simulink model "bus_roadtest_v3"  (R2018a)
settings: Solver=ode3  StartTime=0.0  StopTime=inf  FixedStep=0.01  RelTol=1e-3  EnableMultiTasking=on
PostLoadFcn:
  | , if any(exist('dsrtsu_mdlpostloadfcn', 'file') == [2, 3, 6]), try dsrtsu_mdlpostloadfcn('Execute', bdroot); catch fprintf('Error in PostLoadFcn (dsrtsu_mdlpostloadfcn) for model "%s":\n %s\n', bdroot, lasterr); end, end,
InitFcn:
  | bus_roadtest_v3_initial
values from neighbouring files (symbols this model uses):
  ay_max = 2    [Ini.m]
  delta_t = 0.01    [Ini.m]
  end_left_pass = 1    [Ini.m]
  end_right_pass = 0    [Ini.m]
  finish_node_id = length(Map_data(:,1))    [Ini.m]
  forward_length = 15    [Ini.m]
  gamma = sqrt(N_xaug+lambda)    [bus_roadtest_v3_initial.m]
  k_safe = 1    [Ini.m]
  nodes = nodes(1:index_node,:)    [Ini.m]
  rmin = 10    [Ini.m]
  segments = zeros(length(xy_ends_Pos(:,1)),3)    [Ini.m]
  start_node_id = 1    [Ini.m]
  Ts = 0.01    [bus_roadtest_v3_initial.m]
  Veh_CG = [0.5, 0.2]    [Ini.m]
  Veh_size = [1.99986,6.09558]    [Ini.m]
  vmax = 6    [Ini.m]
  weight = [weight_0,weight_0_cov,weight_i]    [bus_roadtest_v3_initial.m]
undefined symbols (not defined in the file or in its folder): Brake_table, DiscIntNeverNeededParam, Map_data, R, REF_GPS_RFS, Steer_gain_table, T
libraries: rtican x71, simulink x26, rti1401lib_adc_type4 x8, rti1401lib_dio_type4 x1
(part 14 of 18)

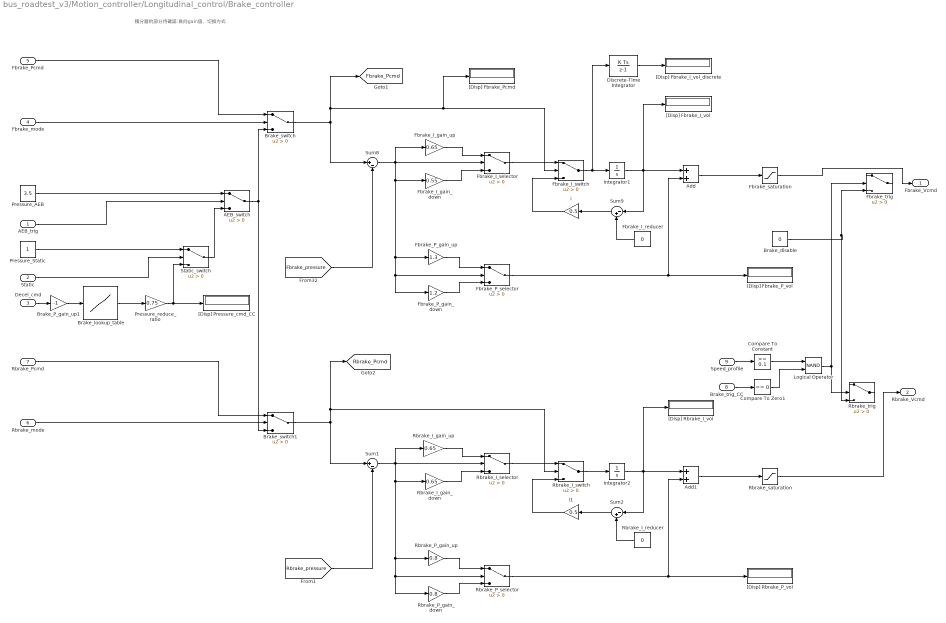
== system bus_roadtest_v3/Motion_controller/Longitudinal_control/Brake_controller ==
  note: 積分器的部分待確認:負向gain值、切換方式
  AEB_trig : Inport
  Static : Inport  Port=2
  Decel_cmd : Inport  Port=3
  Fbrake_mode : Inport  Port=4
  Fbrake_Pcmd : Inport  Port=5
  Rbrake_mode : Inport  Port=6
  Rbrake_Pcmd : Inport  Port=7
  Brake_trig_CC : Inport  Port=8
  Speed_profile : Inport  Port=9
  AEB_switch : Switch  Criteria=u2 > Threshold
  Add : Sum
  Add1 : Sum
  Brake_P_gain_up1 : Gain  Gain=-1
  Brake_disable : Constant  Value=0
  Brake_lookup_table : Lookup_n-D  NumberOfTableDimensions=1  BreakpointsForDimension1=Brake_table(2,:)  Table=Brake_table(1,:)  InterpMethod=Flat  InternalRulePriority=Speed  RndMeth=Simplest  InputSameDT=on
  Brake_switch : Switch  Criteria=u2 > Threshold
  Brake_switch1 : Switch  Criteria=u2 > Threshold
  Compare To Constant : simulink/Logic and Bit Operations/Compare To Constant  relop=>=  const=0.1  OutDataTypeStr=boolean
  Compare To Zero1 : simulink/Logic and Bit Operations/Compare To Zero  relop===  OutDataTypeStr=boolean
  Discrete-Time Integrator : DiscreteIntegrator  SampleTime=0.01  LimitOutput=on  UpperSaturationLimit=5  LowerSaturationLimit=-100  ICPrevOutput=DiscIntNeverNeededParam  ICPrevScaledInput=DiscIntNeverNeededParam
  Fbrake_I_gain_down : Gain  Gain=0.55
  Fbrake_I_gain_up : Gain  Gain=0.65
  Fbrake_I_reducer : Constant  Value=0
  Fbrake_I_selector : Switch  Criteria=u2 > Threshold
  Fbrake_I_switch : Switch  Criteria=u2 > Threshold
  Fbrake_P_gain_down : Gain  Gain=1.2
  Fbrake_P_gain_up : Gain  Gain=1.3
  Fbrake_P_selector : Switch  Criteria=u2 > Threshold
  Fbrake_saturation : Saturate  UpperLimit=4.8  LowerLimit=0
  Fbrake_trig : Switch  Criteria=u2 > Threshold
  Integrator1 : Integrator  LimitOutput=on  UpperSaturationLimit=5  LowerSaturationLimit=-100
  Integrator2 : Integrator  LimitOutput=on  UpperSaturationLimit=5  LowerSaturationLimit=-100
  Logical Operator : Logic  Operator=NAND  AllPortsSameDT=off  OutDataTypeStr=boolean
  Pressure_AEB : Constant  Value=3.5
  Pressure_Static : Constant
  Pressure_reduce_ratio : Gain  Gain=0.75
  Rbrake_I_gain_down : Gain  Gain=0.65
  Rbrake_I_gain_up : Gain  Gain=0.65
  Rbrake_I_reducer : Constant  Value=0
  Rbrake_I_selector : Switch  Criteria=u2 > Threshold
  Rbrake_I_switch : Switch  Criteria=u2 > Threshold
  Rbrake_P_gain_down : Gain  Gain=0.8
  Rbrake_P_gain_up : Gain  Gain=0.8
  Rbrake_P_selector : Switch  Criteria=u2 > Threshold
  Rbrake_saturation : Saturate  UpperLimit=4.8  LowerLimit=0
  Rbrake_trig : Switch  Criteria=u2 > Threshold
  Static_switch : Switch  Criteria=u2 > Threshold
  Sum1 : Sum  Inputs=|+-
  Sum2 : Sum  Inputs=|-+
  Sum8 : Sum  Inputs=|+-
  Sum9 : Sum  Inputs=|-+
  "[Disp] Fbrake_I_vol" : Display
  "[Disp] Fbrake_I_vol_discrete" : Display
  "[Disp] Fbrake_P_vol" : Display
  "[Disp] Fbrake_Pcmd" : Display
  "[Disp] Pressure_cmd_CC" : Display
  "[Disp] Rbrake_I_vol" : Display
  "[Disp] Rbrake_P_vol" : Display
  i : Gain  Gain=0.5
  i1 : Gain  Gain=0.5
  Fbrake_Vcmd : Outport
  Rbrake_Vcmd : Outport  Port=2
  tag scope: Fbrake_Pcmd=global, Rbrake_Pcmd=global
  wires:
  Fbrake_I_gain_up/1 -> Fbrake_I_selector/1
  Fbrake_P_selector/1 -> "[Disp] Fbrake_P_vol"/1, Add/2
  Integrator1/1 -> Add/1, "[Disp] Fbrake_I_vol"/1, Sum9/1
  Sum8/1 -> Fbrake_I_gain_up/1, Fbrake_I_selector/2, Fbrake_P_selector/2, Fbrake_P_gain_down/1, Fbrake_P_gain_up/1, Fbrake_I_gain_down/1
  Fbrake_I_gain_down/1 -> Fbrake_I_selector/3
  Fbrake_P_gain_up/1 -> Fbrake_P_selector/1
  Fbrake_P_gain_down/1 -> Fbrake_P_selector/3
  AEB_trig/1 -> AEB_switch/2
  Pressure_AEB/1 -> AEB_switch/1
  Static_switch/1 -> AEB_switch/3
  Pressure_Static/1 -> Static_switch/1
  Brake_lookup_table/1 -> Pressure_reduce_ratio/1
  [Fbrake_pressure] -> Sum8/2
  Fbrake_I_reducer/1 -> Sum9/2
  Sum9/1 -> i/1
  Fbrake_I_switch/1 -> Discrete-Time Integrator/1, Integrator1/1
  Fbrake_I_selector/1 -> Fbrake_I_switch/1
  i/1 -> Fbrake_I_switch/3
  Decel_cmd/1 -> Brake_P_gain_up1/1
  Brake_P_gain_up1/1 -> Brake_lookup_table/1
  Static/1 -> Static_switch/2
  Fbrake_mode/1 -> Brake_switch/2
  Brake_switch/1 -> [Fbrake_Pcmd], "[Disp] Fbrake_Pcmd"/1, Fbrake_I_switch/2, Sum8/1
  Fbrake_Pcmd/1 -> Brake_switch/1
  Rbrake_Pcmd/1 -> Brake_switch1/1
  Brake_switch1/1 -> Sum1/1, [Rbrake_Pcmd], Rbrake_I_switch/2
  Rbrake_mode/1 -> Brake_switch1/2
  i1/1 -> Rbrake_I_switch/3
  Rbrake_I_selector/1 -> Rbrake_I_switch/1
  Rbrake_I_switch/1 -> Integrator2/1
  Sum2/1 -> i1/1
  Rbrake_I_reducer/1 -> Sum2/2
  [Rbrake_pressure] -> Sum1/2
  Rbrake_P_gain_down/1 -> Rbrake_P_selector/3
  Rbrake_P_gain_up/1 -> Rbrake_P_selector/1
  Rbrake_I_gain_down/1 -> Rbrake_I_selector/3
  Sum1/1 -> Rbrake_I_gain_down/1, Rbrake_P_gain_up/1, Rbrake_P_gain_down/1, Rbrake_P_selector/2, Rbrake_I_selector/2, Rbrake_I_gain_up/1
  Integrator2/1 -> Sum2/1, "[Disp] Rbrake_I_vol"/1, Add1/1
  Rbrake_P_selector/1 -> Add1/2, "[Disp] Rbrake_P_vol"/1
  Rbrake_I_gain_up/1 -> Rbrake_I_selector/1
  Add/1 -> Fbrake_saturation/1
  Add1/1 -> Rbrake_saturation/1
  AEB_switch/1 -> Brake_switch1/3, Brake_switch/3
  Pressure_reduce_ratio/1 -> "[Disp] Pressure_cmd_CC"/1, Static_switch/3
  Brake_disable/1 -> Rbrake_trig/3, Fbrake_trig/3
  Speed_profile/1 -> Compare To Constant/1
  Brake_trig_CC/1 -> Compare To Zero1/1
  Compare To Constant/1 -> Logical Operator/1
  Compare To Zero1/1 -> Logical Operator/2
  Logical Operator/1 -> Fbrake_trig/2, Rbrake_trig/2
  Discrete-Time Integrator/1 -> "[Disp] Fbrake_I_vol_discrete"/1
  Rbrake_saturation/1 -> Rbrake_Vcmd/1
  Fbrake_saturation/1 -> Fbrake_Vcmd/1

== system bus_roadtest_v3/Motion_controller/Longitudinal_control/Switching_module ==
  AEB_trig : Inport
  Static : Inport  Port=2
  Speed_profile : Inport  Port=3
  Brake_trig_CC_status : Inport  Port=4
  Base_decel : Constant  Value=0.2
  Brake_Throttle_toggle : MATLAB Function  TreatAsAtomicUnit=on
  Brake_lock_on : Constant
  Brake_status : MATLAB Function  TreatAsAtomicUnit=on
  Brake_trig_bound : Saturate  UpperLimit=-0.2  LowerLimit=-5
  Brake_trig_shreshold : simulink/Logic and Bit Operations/Compare To Constant  relop=<=  const=-0.8  OutDataTypeStr=boolean
  Compare To Constant : simulink/Logic and Bit Operations/Compare To Constant  relop=>=  const=0.5  OutDataTypeStr=boolean
  Compare To Constant1 : simulink/Logic and Bit Operations/Compare To Constant  relop=>=  const=0.5  OutDataTypeStr=boolean
  Constant : Constant  Value=0
  Constant1 : Constant  Value=100
  Constant2 : Constant  Value=10
  Constant3 : Constant  Value=0.25
  Constant4 : Constant  Value=0.2
  Discrete Transfer Fcn : DiscreteTransferFcn  Numerator=[0.09516]  Denominator=[1 -0.9048]
  Logical Operator : Logic  Operator=OR  Inputs=4  AllPortsSameDT=off  OutDataTypeStr=boolean
  Logical Operator1 : Logic  Operator=OR  AllPortsSameDT=off  OutDataTypeStr=boolean
  Logical Operator2 : Logic  Operator=OR  AllPortsSameDT=off  OutDataTypeStr=boolean
  Logical Operator3 : Logic  AllPortsSameDT=off  OutDataTypeStr=boolean
  MATLAB Function : MATLAB Function  TreatAsAtomicUnit=on
  Relational Operator : RelationalOperator  Operator=>  OutDataTypeStr=boolean  RndMeth=Simplest
  Speed_err_gain : Gain
  Sum : Sum  Inputs=|+-
  Sum1 : Sum  Inputs=|+-
  Switch : Switch  Criteria=u2 > Threshold
  Switch1 : Switch  Criteria=u2 > Threshold
  Switch2 : Switch  Criteria=u2 > Threshold
  Transfer Fcn : TransferFcn  Numerator=[10]  Denominator=[1 10]
  "[Disp] Accel_err" : Display
  "[Disp] Accel_err_discrete" : Display
  "[Disp] Brake_status" : Display
  "[Disp] Brake_trig_CC" : Display
  "[Disp] Decel_cmd" : Display
  "[Disp] Speed_err" : Display
  "[Disp] Throttle_resume" : Display
  kph2mps : Gain  Gain=1/3.6
  Speed_cmd : Outport
  Decel_cmd : Outport  Port=2
  Brake_trig_CC : Outport  Port=3
  tag scope: Brake_status=global, Brake_trig_CC=global
  wires:
  Speed_profile/1 -> Sum/1, Switch/3
  [Speed_Kph] -> MATLAB Function/1(Speed_cmd), Sum/2
  Sum/1 -> kph2mps/1
  kph2mps/1 -> Speed_err_gain/1, "[Disp] Speed_err"/1
  Brake_Throttle_toggle/1(Brake_trig_CC) -> Logical Operator/3, Switch1/2, Brake_status/3(CC_trig), Brake_trig_CC/1, [Brake_trig_CC], "[Disp] Brake_trig_CC"/1
  Brake_trig_shreshold/1 -> Brake_Throttle_toggle/1(B_toggle)
  Relational Operator/1 -> Brake_Throttle_toggle/2(T_toggle)
  Brake_trig_CC_status/1 -> Brake_Throttle_toggle/3(Last_status)
  Switch/1 -> Speed_cmd/1
  Constant/1 -> Switch1/3, Switch/1
  AEB_trig/1 -> Logical Operator/1, Brake_status/1(AEB), Logical Operator1/1
  Static/1 -> Brake_status/2(Static), Logical Operator/2, Logical Operator1/2, Brake_Throttle_toggle/4(Static_flag)
  Logical Operator/1 -> Switch/2
  Switch2/1 -> "[Disp] Decel_cmd"/1, Decel_cmd/1
  Logical Operator1/1 -> Switch2/2
  Switch1/1 -> Switch2/3
  Constant1/1 -> Switch2/1
  Speed_err_gain/1 -> Discrete Transfer Fcn/1, Transfer Fcn/1
  Sum1/1 -> Brake_trig_bound/1
  Transfer Fcn/1 -> "[Disp] Accel_err"/1, Sum1/1, Relational Operator/1, Brake_trig_shreshold/1
  Base_decel/1 -> Sum1/2
  Brake_trig_bound/1 -> Switch1/1
  Constant2/1 -> MATLAB Function/2(Speed_bound)
  Constant3/1 -> MATLAB Function/3(upper_ratio)
  Constant4/1 -> MATLAB Function/4(lower_ratio)
  MATLAB Function/1(T_resume) -> "[Disp] Throttle_resume"/1, Relational Operator/2
  [Fbrake_pressure] -> Compare To Constant/1
  [Rbrake_pressure] -> Compare To Constant1/1
  Compare To Constant1/1 -> Logical Operator2/2
  Compare To Constant/1 -> Logical Operator2/1
  Logical Operator2/1 -> Logical Operator3/2
  Logical Operator3/1 -> Logical Operator/4
  Brake_lock_on/1 -> Logical Operator3/1
  Discrete Transfer Fcn/1 -> "[Disp] Accel_err_discrete"/1
  [Fbrake_interrupt] -> Brake_status/4(interrupt)
  Brake_status/1(Brake_status) -> [Brake_status], "[Disp] Brake_status"/1

== system bus_roadtest_v3/Motion_controller/Longitudinal_control/Throttle_controller ==
  Throttle_mode : Inport
  Throttle_vol : Inport  Port=2
  AEB_trig : Inport  Port=3
  Static : Inport  Port=4
  Speed_cmd : Inport  Port=5
  AEB_switch_T : Switch  Criteria=u2 > Threshold
  Constant : Constant  Value=0
  I_gain_windup : Switch  Criteria=u2 > Threshold
  I_gain_windup1 : Switch  Criteria=u2 > Threshold
  I_windup_limit : simulink/Logic and Bit Operations/Compare To Constant  relop=<=  const=2  OutDataTypeStr=boolean
  I_windup_on : Constant
  Logical Operator : Logic  Operator=OR  AllPortsSameDT=off  OutDataTypeStr=boolean
  Sum1 : Sum  Inputs=|++
  Sum2 : Sum  Inputs=|+-
  Sum3 : Sum  Inputs=|+-
  Sum4 : Sum  Inputs=+|+
  Sum6 : Sum  Inputs=|++
  Sum7 : Sum  Inputs=|+-
  Throttle_I_gain : Gain  Gain=0.05
  Throttle_I_gain_down : Gain  Gain=0.05
  Throttle_I_integrator : Integrator  LimitOutput=on  UpperSaturationLimit=4.68  LowerSaturationLimit=0
  Throttle_I_reducer : Constant  Value=0
  Throttle_I_saturation : Saturate  UpperLimit=2  LowerLimit=0
  Throttle_I_switch : Switch  Criteria=u2 > Threshold
  Throttle_I_switch1 : Switch  Criteria=u2 > Threshold
  Throttle_P_gain : Gain  Gain=0.2
  Throttle_boost_on : Constant
  Throttle_boost_vol : Constant  Value=0.8
  Throttle_boost_zero : Constant  Value=0
  Throttle_saturation : Saturate  UpperLimit=4.68  LowerLimit=0.04
  Throttle_switch : Switch  Criteria=u2 > Threshold
  Throttle_switch1 : Switch  Criteria=u2 > Threshold
  Throttle_switch2 : Switch  Criteria=u2 > Threshold
  "[Disp] Speed_cmd_controller" : Display
  "[Disp] Throttle_I_vol" : Display
  "[Disp] Throttle_I_windup" : Display
  "[Disp] Throttle_P_vol" : Display
  "[Disp] Throttle_T_vol" : Display
  "[Disp] Throttle_boost_vol" : Display
  speed P gain1 : Gain  Gain=0.5
  Throttle_out : Outport
  wires:
  Throttle_vol/1 -> Throttle_switch/1
  Sum2/1 -> Throttle_P_gain/1, Throttle_I_gain_down/1, Throttle_I_switch1/2, Throttle_I_gain/1
  Throttle_P_gain/1 -> "[Disp] Throttle_P_vol"/1, Sum6/1
  Throttle_I_integrator/1 -> Sum3/2, Sum7/2, Throttle_I_saturation/1, Sum6/2, "[Disp] Throttle_I_vol"/1
  Throttle_I_switch/1 -> Throttle_I_integrator/1
  Throttle_I_reducer/1 -> Sum7/1, I_gain_windup1/3, I_gain_windup/1
  Sum7/1 -> speed P gain1/1
  speed P gain1/1 -> Throttle_I_switch/3
  Throttle_saturation/1 -> "[Disp] Throttle_T_vol"/1, Throttle_switch/3
  Speed_cmd/1 -> Sum2/1, "[Disp] Speed_cmd_controller"/1, Throttle_switch2/2, Throttle_I_switch/2
  [Speed_Kph] -> Sum2/2
  AEB_trig/1 -> Logical Operator/1
  Static/1 -> Logical Operator/2
  Throttle_switch/1 -> AEB_switch_T/3
  AEB_switch_T/1 -> Throttle_out/1
  Logical Operator/1 -> AEB_switch_T/2
  Constant/1 -> AEB_switch_T/1
  Throttle_mode/1 -> Throttle_switch/2
  Throttle_boost_vol/1 -> Throttle_switch2/1
  Throttle_boost_on/1 -> Throttle_switch1/2
  Throttle_boost_zero/1 -> Throttle_switch2/3, Throttle_switch1/3
  Sum6/1 -> Sum1/1
  Sum1/1 -> Throttle_saturation/1
  Throttle_switch1/1 -> "[Disp] Throttle_boost_vol"/1, Sum1/2
  Throttle_switch2/1 -> Throttle_switch1/1
  Throttle_I_gain/1 -> Throttle_I_switch1/1
  Throttle_I_gain_down/1 -> Throttle_I_switch1/3
  Throttle_I_saturation/1 -> Sum3/1
  Sum3/1 -> I_gain_windup/3
  Throttle_I_switch1/1 -> Sum4/1
  Sum4/1 -> Throttle_I_switch/1
  [Speed_Kph] -> I_windup_limit/1
  I_windup_limit/1 -> I_gain_windup/2
  I_windup_on/1 -> I_gain_windup1/2
  I_gain_windup1/1 -> "[Disp] Throttle_I_windup"/1, Sum4/2
  I_gain_windup/1 -> I_gain_windup1/1

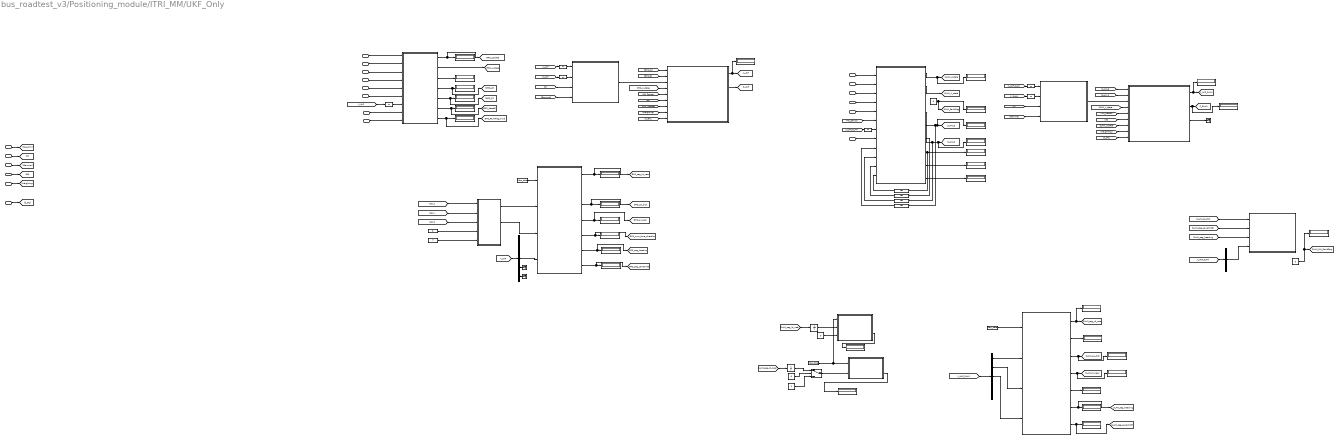
== system bus_roadtest_v3/Positioning_module/ITRI_MM/UKF_Only ==
  note: 建立取樣點UKF(對照組)
  note: 建立取樣點UKF_SLAM
  note: MM線段:得知當下最近道路，得知道路資訊
  note: GNSS模組
  note: GNSS Check
  note: GNSS MM
  note: SLAM模組
  note: SLAM Check
  note: SLAM UKF
  note: SLAM UKF MM
  note: SLAM UKF MM Check模組
  GPS_X : Inport
  GPS_Y : Inport  Port=2
  GPS_Heading : Inport  Port=3
  Road _Alt_GPS : Inport  Port=4
  IMU : Inport  Port=5
  Sig_dim : Inport  Port=6
  N : Inport  Port=7
  Gamma : Inport  Port=8
  dt : Inport  Port=9
  weighting : Inport  Port=10
  GPS_TYPE : Inport  Port=11
  GPS_X_ACC : Inport  Port=12
  GPS_Y_ACC : Inport  Port=13
  d_GC : Inport  Port=14
  SLAM_X : Inport  Port=15
  SLAM_Y : Inport  Port=16
  SLAM_Heading : Inport  Port=17
  SLAM_Counter : Inport  Port=18
  SLAM_FS : Inport  Port=19
  SLAM_fault : Inport  Port=20
  Constant : Constant  Value=0
  Constant1 : Constant  Value=Map_data
  Constant2 : Constant  Value=T
  Constant22 : Constant  Value=Map_data
  Constant29 : Constant  Value=R
  Constant3 : Constant  Value=0
  Constant4 : Constant  Value=Map_data
  Demux : Demux  Outputs=5
  Demux1 : Demux  Outputs=5
  Demux2 : Demux  Outputs=5
  ENU2SLAM : MATLAB Function  TreatAsAtomicUnit=on
  GNSS_Check : Subsystem
  GNSS_UKF : MATLAB Function  TreatAsAtomicUnit=on
  GNSS_UKF_MM : MATLAB Function  TreatAsAtomicUnit=on
  Generate_sigma_pt_UKF : MATLAB Function  TreatAsAtomicUnit=on
  MATLAB Function : MATLAB Function  TreatAsAtomicUnit=on
  MATLAB Function1 : MATLAB Function  TreatAsAtomicUnit=on
  SLAM_Check : MATLAB Function  TreatAsAtomicUnit=on
  SLAM_Generate_sigma_pt_UKF : MATLAB Function  TreatAsAtomicUnit=on
  SLAM_UKF : MATLAB Function  TreatAsAtomicUnit=on
  SLAM_UKF_MM : MATLAB Function  TreatAsAtomicUnit=on
  SLAM_UKF_MM_Check : MATLAB Function  TreatAsAtomicUnit=on
  Switch : Switch  Criteria=u2 > Threshold
  Terminator2 : Terminator
  Terminator3 : Terminator
  Terminator5 : Terminator
  Unit Delay : UnitDelay  InitialCondition=1  SampleTime=-1
  Unit Delay{1,9,14,34} (4 alike) : UnitDelay  InitialCondition=[0;0;0;0;0]  SampleTime=-1
  Unit Delay10 : UnitDelay  InitialCondition=[eye(5)*0.001]  SampleTime=-1
  Unit Delay2 : UnitDelay  InitialCondition=1  SampleTime=-1
  Unit Delay33 : UnitDelay  InitialCondition=[eye(5)*0.001]  SampleTime=-1
  Unit Delay35 : UnitDelay  InitialCondition=[0,0,0,0]  SampleTime=-1
  Unit Delay36 : UnitDelay  InitialCondition=diag([0.1,0.1,0.1,0.0001,0.0001])  SampleTime=-1
  Unit Delay37 : UnitDelay  InitialCondition=diag([0.00025,0.00025,0.0000001,1,0.0001])  SampleTime=-1
  Unit Delay38 : UnitDelay  SampleTime=-1
  "[Disp] Forward_segid" : Display
  "[Disp] Forward_segid1" : Display
  "[Disp] GPS_FaultFlag" : Display
  "[Disp] GPS_FaultFlag_True" : Display
  "[Disp] GPS_Q" : Display
  "[Disp] GPS_R" : Display
  "[Disp] GPS_ResetP" : Display
  "[Disp] GPS_Update_UKF" : Display
  "[Disp] GPS_num_lane_direction" : Display
  "[Disp] GPS_oi_near" : Display
  "[Disp] GPS_op_dist" : Display
  "[Disp] GPS_seg_LaneWidth" : Display
  "[Disp] GPS_seg_heading" : Display
  "[Disp] GPS_seg_id_near" : Display
  "[Disp] P_SLAM" : Display
  "[Disp] SLAM_FaultFalg" : Display
  "[Disp] SLAM_FaultFlag_case" : Display
  "[Disp] SLAM_MM_FaultFlag" : Display
  "[Disp] SLAM_Q" : Display
  "[Disp] SLAM_R" : Display
  "[Disp] SLAM_dist_op" : Display
  "[Disp] SLAM_num_lane_direction" : Display
  "[Disp] SLAM_oi_near" : Display
  "[Disp] SLAM_op_dist" : Display
  "[Disp] SLAM_seg_LaneWidth" : Display
  "[Disp] SLAM_seg_heading" : Display
  "[Disp] SLAM_seg_id_near" : Display
  "[Disp] SLAM_update" : Display
  "[Disp] SLAM_update_count" : Display
  "[Disp] X_UKF" : Display
  "[Disp] X_UKF_SLAM" : Display
  "[Disp] dist_SLAMlastUKFSLAM" : Display
  "[Para] Inisegid" : Constant
  "[Para] Inisegswitch" : Constant  Value=0
  "[Para] Map_switch" : Constant  Value=0
  tag scope: GPS_FaultFlag_True=global, GPS_Update=global, GPS_X_state=global, GPS_num_lane_direction=global, GPS_oi_near=global, GPS_op_dist=global, GPS_seg_LaneWidth=global, GPS_seg_heading=global, GPS_seg_id_near=global, P_SLAM=global, P_UKF=global, SLAM_FaultFlag=global, SLAM_MM_FaultFlag=global, SLAM_Q=global, SLAM_R=global, SLAM_X_state=global, SLAM_oi_near=global, SLAM_op_dist=global, SLAM_seg_LaneWidth=global, SLAM_seg_heading=global, SLAM_seg_id_near=global, SLAM_update=global, X_UKF=global, X_UKF_SLAM=global
  wires:
  GNSS_Check/1(GPS_update) -> [GPS_Update], "[Disp] GPS_Update_UKF"/1
  GNSS_Check/2(X_state) -> [GPS_X_state]
  Sig_dim/1 -> [Sig_dim]
  N/1 -> [N]
  Gamma/1 -> [Gamma]
  dt/1 -> [dt]
  weighting/1 -> [weighting]
  Unit Delay10/1 -> Generate_sigma_pt_UKF/2(IC_P)
  Unit Delay9/1 -> Generate_sigma_pt_UKF/1(IC_X)
  [X_UKF] -> Unit Delay9/1
  [P_UKF] -> Unit Delay10/1
  [N] -> Generate_sigma_pt_UKF/3(n)
  [Gamma] -> Generate_sigma_pt_UKF/4(gamma)
  GPS_X/1 -> GNSS_Check/1(GPS_X)
  GPS_Y/1 -> GNSS_Check/2(GPS_Y)
  GPS_Heading/1 -> GNSS_Check/3(GPS_Heading)
  Road _Alt_GPS/1 -> GNSS_Check/4(Road_Alt_GPS)
  IMU/1 -> GNSS_Check/5(IMU)
  GPS_TYPE/1 -> GNSS_Check/6(GPS_TYPE)
  GNSS_Check/4(Q_last_o) -> [GPS_Q], "[Disp] GPS_Q"/1
  GNSS_Check/5(R_last_o) -> [GPS_R], "[Disp] GPS_R"/1
  [X_UKF] -> Unit Delay14/1
  Unit Delay14/1 -> GNSS_Check/7(X_UKF)
  GNSS_Check/3(GNSS_FaultFlag) -> "[Disp] GPS_FaultFlag"/1
  GNSS_Check/6(ResetP) -> [GPS_ResetP], "[Disp] GPS_ResetP"/1
  GPS_X_ACC/1 -> GNSS_Check/8(GPS_X_Acc)
  GPS_Y_ACC/1 -> GNSS_Check/9(GPS_Y_Acc)
  d_GC/1 -> [d_GC]
  [X_UKF] -> Demux/1
  Demux/4 -> Terminator2/1
  Demux/5 -> Terminator3/1
  [N] -> SLAM_Generate_sigma_pt_UKF/3(n)
  [Gamma] -> SLAM_Generate_sigma_pt_UKF/4(gamma)
  SLAM_Generate_sigma_pt_UKF/1(X_AUG) -> SLAM_UKF/3(X_AUG)
  [SLAM_X_state] -> SLAM_UKF/4(X_state)
  [SLAM_update] -> SLAM_UKF/7(SLAM_update)
  [dt] -> SLAM_UKF/6(Sensor_dt)
  [IMU_Sensor] -> SLAM_UKF/5(IMU_Sensor)
  [weighting] -> SLAM_UKF/8(weighting)
  SLAM_UKF/1(X) -> "[Disp] X_UKF_SLAM"/1, [X_UKF_SLAM]
  SLAM_UKF/2(P) -> "[Disp] P_SLAM"/1, [P_SLAM]
  SLAM_UKF/3(K) -> Terminator5/1
  Unit Delay33/1 -> SLAM_Generate_sigma_pt_UKF/2(IC_P)
  Unit Delay34/1 -> SLAM_Generate_sigma_pt_UKF/1(IC_X)
  [X_UKF_SLAM] -> Unit Delay34/1
  [P_SLAM] -> Unit Delay33/1
  SLAM_UKF_MM/3(op_distance) -> "[Disp] SLAM_op_dist"/1, [SLAM_op_dist]
  SLAM_UKF_MM/1(seg_id_near) -> "[Disp] SLAM_seg_id_near"/1, [SLAM_seg_id_near]
  SLAM_UKF_MM/4(Oi_near) -> "[Disp] SLAM_oi_near"/1, [SLAM_oi_near]
  [SLAM_R] -> SLAM_UKF/2(R)
  SLAM_UKF_MM/5(num_lane_direction) -> "[Disp] SLAM_num_lane_direction"/1
  [SLAM_Q] -> SLAM_UKF/1(Q)
  [d_GC] -> SLAM_UKF/9(d_GC)
  SLAM_X/1 -> SLAM_Check/2(SLAM_X)
  SLAM_Y/1 -> SLAM_Check/3(SLAM_Y)
  SLAM_Heading/1 -> SLAM_Check/4(SLAM_Heading)
  SLAM_Counter/1 -> SLAM_Check/5(SLAM_Counter)
  [IMU_Sensor] -> SLAM_Check/6(IMU_Sensor)
  SLAM_FS/1 -> SLAM_Check/8(SLAM_FS)
  SLAM_Check/1(SLAM_update) -> "[Disp] SLAM_update"/1, [SLAM_update]
  SLAM_Check/2(X_state) -> [SLAM_X_state]
  SLAM_Check/4(Q_last_o) -> Unit Delay37/1, "[Disp] SLAM_Q"/1, [SLAM_Q]
  SLAM_Check/5(R_last_o) -> Unit Delay36/1, "[Disp] SLAM_R"/1, [SLAM_R]
  SLAM_Check/6(Last_SLAM_Out) -> Unit Delay35/1
  Unit Delay35/1 -> SLAM_Check/11(Last_SLAM_In)
  Unit Delay36/1 -> SLAM_Check/10(R_last_i)
  Unit Delay37/1 -> SLAM_Check/9(Q_last_i)
  SLAM_fault/1 -> SLAM_Check/1(SLAM_fault)
  SLAM_Check/7(count_o) -> "[Disp] SLAM_update_count"/1, Unit Delay38/1
  Unit Delay38/1 -> SLAM_Check/12(count_i)
  [X_UKF_SLAM] -> Unit Delay1/1
  Unit Delay1/1 -> SLAM_Check/7(X_UKF)
  [X_UKF_SLAM] -> Demux1/1
  Demux1/1 -> SLAM_UKF_MM/2(Position_X)
  Demux1/2 -> SLAM_UKF_MM/3(Postion_Y)
  Demux1/3 -> SLAM_UKF_MM/4(Position_H)
  SLAM_UKF_MM/6(seg_heading) -> [SLAM_seg_heading], "[Disp] SLAM_seg_heading"/1
  SLAM_UKF_MM/7(seg_LaneWidth) -> "[Disp] SLAM_seg_LaneWidth"/1, [SLAM_seg_LaneWidth]
  [X_UKF_SLAM] -> Demux2/1
  Demux2/3 -> SLAM_UKF_MM_Check/4(X_UKF_SLAM_heading)
  [SLAM_seg_heading] -> SLAM_UKF_MM_Check/3(SLAM_seg_heading)
  [SLAM_seg_LaneWidth] -> SLAM_UKF_MM_Check/2(SLAM_seg_LaneWidth)
  [SLAM_op_dist] -> SLAM_UKF_MM_Check/1(SLAM_op_dist)
  GNSS_Check/7(GNSS_FaultFlag_True) -> [GPS_FaultFlag_True], "[Disp] GPS_FaultFlag_True"/1
  GNSS_UKF/1(X) -> "[Disp] X_UKF"/1, [X_UKF]
  [GPS_Q] -> GNSS_UKF/1(Q)
  [GPS_R] -> GNSS_UKF/2(R)
  [GPS_X_state] -> GNSS_UKF/4(X_state)
  [IMU_Sensor] -> GNSS_UKF/5(IMU_Sensor)
  [dt] -> GNSS_UKF/6(Sensor_dt)
  [GPS_Update] -> GNSS_UKF/7(GNSS_update)
  [weighting] -> GNSS_UKF/8(weighting)
  [d_GC] -> GNSS_UKF/9(d_GC)
  Generate_sigma_pt_UKF/1(X_AUG) -> GNSS_UKF/3(X_AUG)
  GNSS_UKF/2(P) -> [P_UKF]
  Constant1/1 -> GNSS_UKF_MM/1(Map_data)
  GNSS_UKF_MM/1(seg_id_near) -> [GPS_seg_id_near], "[Disp] GPS_seg_id_near"/1
  GNSS_UKF_MM/7(seg_LaneWidth) -> [GPS_seg_LaneWidth], "[Disp] GPS_seg_LaneWidth"/1
  GNSS_UKF_MM/6(seg_heading) -> [GPS_seg_heading], "[Disp] GPS_seg_heading"/1
  GNSS_UKF_MM/4(Oi_near) -> [GPS_oi_near], "[Disp] GPS_oi_near"/1
  GNSS_UKF_MM/3(op_distance) -> [GPS_op_dist], "[Disp] GPS_op_dist"/1
  GNSS_UKF_MM/5(num_lane_direction) -> [GPS_num_lane_direction], "[Disp] GPS_num_lane_direction"/1
  Demux/3 -> GNSS_UKF_MM/4(Position_H)
  ENU2SLAM/1(Car_SLAM_x) -> GNSS_UKF_MM/2(Position_X)
  ENU2SLAM/2(Car_SLAM_y) -> GNSS_UKF_MM/3(Postion_Y)
  [Car_X] -> ENU2SLAM/1(Car_x)
  [Car_Y] -> ENU2SLAM/2(Car_y)
  [Car_Z] -> ENU2SLAM/3(Car_z)
  Constant2/1 -> ENU2SLAM/5(T)
  Constant29/1 -> ENU2SLAM/4(R)
  SLAM_Check/8(dist_SLAMlastUKFSLAM) -> "[Disp] dist_SLAMlastUKFSLAM"/1
  SLAM_Check/9(SLAM_FaultFlag_case) -> "[Disp] SLAM_FaultFlag_case"/1
  Constant/1 -> "[Disp] SLAM_MM_FaultFlag"/1, [SLAM_MM_FaultFlag]
  Constant3/1 -> "[Disp] SLAM_FaultFalg"/1, [SLAM_FaultFlag]
  Constant22/1 -> MATLAB Function1/1(Map_data), MATLAB Function/1(Map_data)
  [SLAM_seg_id_near] -> Unit Delay/1
  MATLAB Function/2(forward_segid) -> "[Disp] Forward_segid"/1
  "[Para] Inisegid"/1 -> Switch/3
  Switch/1 -> MATLAB Function/2(seg_id_near)
  Unit Delay/1 -> Switch/1
  "[Para] Inisegswitch"/1 -> Switch/2
  SLAM_UKF_MM/2(dist_op) -> "[Disp] SLAM_dist_op"/1
  Unit Delay2/1 -> MATLAB Function1/2(seg_id_near)
  MATLAB Function1/2(forward_segid) -> "[Disp] Forward_segid1"/1
  [SLAM_seg_id_near] -> Unit Delay2/1
  "[Para] Map_switch"/1 -> MATLAB Function1/3(Map_switch)
  Constant4/1 -> SLAM_UKF_MM/1(Map_data)

== system bus_roadtest_v3/RTI Data/RTI Data Store/RTI Data Store ==
  RTI Data Store : Subsystem  mask(RTI_DATA_STORE){}
      mask help:
      | RTI Data Store Block. This block is used by RTI to store internal model dependent data. Deleting this block will result in data loss.
      |
      | NEVER DELETE, COPY, OR MODIFY THIS BLOCK!
      mask Help:
      | RTI Data Store Block. This block is used by RTI to store internal model dependent data. Deleting this block will result in data loss.
      | 
      | NEVER DELETE, COPY, OR MODIFY THIS BLOCK!
      mask Display: text(0.5, 0.5, ' ', 'HorizontalAlignment', 'center');

== system bus_roadtest_v3/Speed_profile/High level controller/ACC ==
  Ego_speed : Inport
  Front_abs_speed : Inport  Port=2
  Rel_distance : Inport  Port=3
  Speed_set : Inport  Port=4
  Add1 : Sum
  Constant2 : Constant  Value=0
  FS_set : Constant  Value=0
  Filter : MATLAB Function  TreatAsAtomicUnit=on
  FrontSpeed_swtich : Constant
  Gain : Gain  Gain=3.6
  "Lowpass_filter " : TransferFcn  Numerator=[10]  Denominator=[1 10]
  MATLAB Function : MATLAB Function  TreatAsAtomicUnit=on
  MATLAB Function1 : MATLAB Function  TreatAsAtomicUnit=on
  Ref_table : Lookup_n-D  NumberOfTableDimensions=1  BreakpointsForDimension1="[0 5 10 15  20]"  Table=[3 3 5 8 11]  InternalRulePriority=Speed  RndMeth=Simplest  InputSameDT=on
  Switch : Switch  Criteria=u2 > Threshold
  "[Disp] Front_speed" : Display
  "[Disp] Front_speed_filtered" : Display
  "[Disp] Reference_m" : Display
  "[Para]Cons_Headway" : Constant  Value=9
  "[Para]Ref_switch" : Constant  Value=0
  switch : Switch  Criteria=u2 > Threshold
  Speed_cmd : Outport
  close_flag : Outport  Port=2
  wires:
  [Reference_m] -> MATLAB Function/2(Reference_m)
  Rel_distance/1 -> [Relative_distance]
  [Relative_distance] -> MATLAB Function/1(Relative_distance)
  Front_abs_speed/1 -> Gain/1
  Speed_set/1 -> [Speed_set]
  [Speed_set] -> MATLAB Function/4(Speed_set)
  Gain/1 -> Filter/1(u), "[Disp] Front_speed"/1
  [AEB_range] -> MATLAB Function/5(AEB_range)
  Ego_speed/1 -> [Ego_speed], Ref_table/1
  Ref_table/1 -> switch/1
  "[Para]Ref_switch"/1 -> switch/2
  "[Para]Cons_Headway"/1 -> switch/3
  FrontSpeed_swtich/1 -> Switch/2
  FS_set/1 -> Switch/3
  Switch/1 -> MATLAB Function/3(Front_speed)
  [Front_speed_kph] -> Switch/1
  MATLAB Function/2(close_flag) -> close_flag/1
  switch/1 -> [Reference_m]
  Filter/1(y) -> "Lowpass_filter "/1
  "Lowpass_filter "/1 -> "[Disp] Front_speed_filtered"/1, [Front_speed_kph]
  [Reference_m] -> Add1/1
  [AEB_range] -> Add1/2
  Add1/1 -> "[Disp] Reference_m"/1
  MATLAB Function/1(cmd) -> MATLAB Function1/1(cmd)
  [Ego_speed] -> MATLAB Function1/2(Ego_speed)
  MATLAB Function1/1(cmd_limited) -> Speed_cmd/1

== system bus_roadtest_v3/Flag_management/Fault detection/Fault detection(Control)/Brake fault detection ==
  In1 : Inport
  In2 : Inport  Port=2
  Add2 : Sum  Inputs=+-
  Compare To Constant : simulink/Logic and Bit Operations/Compare To Constant  relop=<=  const=-8  OutDataTypeStr=boolean
  MATLAB Function1 : MATLAB Function  TreatAsAtomicUnit=on
  MATLAB Function2 : MATLAB Function  TreatAsAtomicUnit=on
  "[Disp] Brake_diff" : Display
  Out1 : Outport
  wires:
  In2/1 -> Add2/2
  In1/1 -> Add2/1
  Compare To Constant/1 -> Out1/1
  Add2/1 -> Compare To Constant/1, "[Disp] Brake_diff"/1, MATLAB Function2/1(u)

== system bus_roadtest_v3/Flag_management/Fault detection/Fault detection(Control)/Speed fault detection ==
  In1 : Inport
  In2 : Inport  Port=2
  Abs : Abs
  Add3 : Sum  Inputs=+-
  Compare To Constant1 : simulink/Logic and Bit Operations/Compare To Constant  relop=>=  const=50  OutDataTypeStr=boolean
  MATLAB Function6 : MATLAB Function  TreatAsAtomicUnit=on
  MATLAB Function7 : MATLAB Function  TreatAsAtomicUnit=on
  Out1 : Outport
  wires:
  Add3/1 -> MATLAB Function6/1(u)
  MATLAB Function6/1(y) -> Abs/1
  Abs/1 -> Compare To Constant1/1
  MATLAB Function7/1(y) -> Add3/1
  In2/1 -> Add3/2
  In1/1 -> MATLAB Function7/1(u)
  Compare To Constant1/1 -> Out1/1

== system bus_roadtest_v3/Flag_management/Fault detection/Fault detection(Control)/Steer fault detection ==
  In1 : Inport
  In2 : Inport  Port=2
  Abs1 : Abs
  Add1 : Sum  Inputs=+-
  Compare To Constant2 : simulink/Logic and Bit Operations/Compare To Constant  relop=>=  const=300  OutDataTypeStr=boolean
  MATLAB Function4 : MATLAB Function  TreatAsAtomicUnit=on
  MATLAB Function5 : MATLAB Function  TreatAsAtomicUnit=on
  Out1 : Outport
  wires:
  In2/1 -> Add1/2
  Add1/1 -> MATLAB Function4/1(u)
  Abs1/1 -> Compare To Constant2/1
  MATLAB Function5/1(y) -> Add1/1
  MATLAB Function4/1(y) -> Abs1/1
  Compare To Constant2/1 -> Out1/1
  In1/1 -> MATLAB Function5/1(u)

== system bus_roadtest_v3/Positioning_module/ITRI_MM/UKF_Only/GNSS_Check ==
  GPS_X : Inport
  GPS_Y : Inport  Port=2
  GPS_Heading : Inport  Port=3
  Road_Alt_GPS : Inport  Port=4
  IMU : Inport  Port=5
  GPS_TYPE : Inport  Port=6
  X_UKF : Inport  Port=7
  GPS_X_Acc : Inport  Port=8
  GPS_Y_Acc : Inport  Port=9
  Multipath_detection : MATLAB Function  TreatAsAtomicUnit=on
  RTK : MATLAB Function  TreatAsAtomicUnit=on
  Switch{,1..5} (6 alike) : Switch  Criteria=u2 > Threshold
  Unit Delay1 : UnitDelay  InitialCondition=[0,0,0]  SampleTime=-1
  Unit Delay10 : UnitDelay  SampleTime=-1
  Unit Delay12 : UnitDelay  InitialCondition=[0,0,0]  SampleTime=-1
  Unit Delay13 : UnitDelay  InitialCondition=6  SampleTime=-1
  Unit Delay2 : UnitDelay  InitialCondition=diag([0.1,0.1,0.1,0.0001,0.0001])  SampleTime=-1
  Unit Delay3 : UnitDelay  InitialCondition=diag([0.0001,0.0001,0.000001,10,0.0001])  SampleTime=-1
  Unit Delay4 : UnitDelay  InitialCondition=[0;0]  SampleTime=-1
  Unit Delay5 : UnitDelay  InitialCondition=[0;0]  SampleTime=-1
  Unit Delay6 : UnitDelay  InitialCondition=diag([0.1,0.1,0.1,0.0001,0.0001])  SampleTime=-1
  Unit Delay7 : UnitDelay  InitialCondition=[0;0]  SampleTime=-1
  Unit Delay8 : UnitDelay  InitialCondition=diag([0.00025,0.00025,0.0000001,1,0.0001])  SampleTime=-1
  Unit Delay9 : UnitDelay  SampleTime=-1
  WithoutRTK : MATLAB Function  TreatAsAtomicUnit=on
  WithoutRTKresetP : Constant  Value=0
  "[Disp] GNSS_FaultFlag_True" : Display
  "[Disp] GPS_update_True" : Display
  "[Para] RTK_or_not" : Constant  Value=0
  GPS_update : Outport
  X_state : Outport  Port=2
  GNSS_FaultFlag : Outport  Port=3
  Q_last_o : Outport  Port=4
  R_last_o : Outport  Port=5
  ResetP : Outport  Port=6
  GNSS_FaultFlag_True : Outport  Port=7
  wires:
  Unit Delay12/1 -> RTK/15(Last_GPS_In)
  RTK/6(Last_GPS_Out) -> Unit Delay12/1
  RTK/5(R_last_o) -> Unit Delay6/1, Switch4/1
  Unit Delay6/1 -> RTK/14(R_last_i)
  RTK/4(Q_last_o) -> Switch3/1, Unit Delay8/1
  Unit Delay8/1 -> RTK/13(Q_last_i)
  Unit Delay1/1 -> WithoutRTK/12(Last_GPS_In)
  WithoutRTK/6(Last_GPS_Out) -> Unit Delay1/1
  WithoutRTK/5(R_last_o) -> Switch4/3, Unit Delay2/1
  Unit Delay2/1 -> WithoutRTK/11(R_last_i)
  WithoutRTK/4(Q_last_o) -> Switch3/3, Unit Delay3/1
  Unit Delay3/1 -> WithoutRTK/10(Q_last_i)
  GPS_X/1 -> Multipath_detection/1(GPS_X), WithoutRTK/1(GPS_X), RTK/3(GPS_X)
  GPS_Y/1 -> Multipath_detection/2(GPS_Y), WithoutRTK/2(GPS_Y), RTK/4(GPS_Y)
  GPS_Heading/1 -> WithoutRTK/3(GPS_Heading), RTK/5(GPS_Heading)
  Road_Alt_GPS/1 -> RTK/6(Road_Alt_GPS), WithoutRTK/4(Road_Alt_GPS)
  IMU/1 -> WithoutRTK/5(IMU_Sensor), RTK/7(IMU_Sensor)
  GPS_TYPE/1 -> WithoutRTK/6(GPS_TYPE), Unit Delay13/1, RTK/8(GPS_TYPE)
  X_UKF/1 -> WithoutRTK/7(X_UKF), RTK/10(X_UKF), Multipath_detection/3(X_UKF)
  Switch/1 -> GPS_update/1
  RTK/1(GPS_update) -> Switch/1
  "[Para] RTK_or_not"/1 -> Switch5/2, Switch4/2, Switch3/2, Switch2/2, Switch1/2, Switch/2
  WithoutRTK/1(GPS_update) -> Switch/3
  Switch1/1 -> X_state/1
  RTK/2(X_state) -> Switch1/1
  WithoutRTK/2(X_state) -> Switch1/3
  Switch2/1 -> GNSS_FaultFlag/1
  RTK/3(GNSS_FaultFlag) -> Switch2/1
  WithoutRTK/3(GNSS_FaultFlag) -> Switch2/3
  Switch3/1 -> Q_last_o/1
  Switch4/1 -> R_last_o/1
  Unit Delay13/1 -> RTK/9(Last_GPS_Type_In)
  Switch5/1 -> ResetP/1
  RTK/7(ResetP) -> Switch5/1
  WithoutRTKresetP/1 -> Switch5/3
  Unit Delay4/1 -> Multipath_detection/6(Last_GPS_In)
  Unit Delay5/1 -> Multipath_detection/7(Last_UKF_In)
  Unit Delay7/1 -> Multipath_detection/8(Last_GPS_est_In)
  Multipath_detection/3(Last_GPS_Out) -> Unit Delay4/1
  Multipath_detection/4(Last_UKF_Out) -> Unit Delay5/1
  Multipath_detection/5(Last_GPS_est_Out) -> Unit Delay7/1
  Multipath_detection/2(GNSS_FaultFlag_True) -> RTK/2(GNSS_FaultFlag_True), GNSS_FaultFlag_True/1, "[Disp] GNSS_FaultFlag_True"/1
  Multipath_detection/1(GPS_update_True) -> RTK/1(GPS_update_True), "[Disp] GPS_update_True"/1
  RTK/8(count_out) -> Unit Delay9/1
  Unit Delay9/1 -> RTK/16(count_in)
  GPS_X_Acc/1 -> WithoutRTK/8(GPS_X_Acc), Multipath_detection/4(GPS_X_Acc), RTK/11(GPS_X_Acc)
  GPS_Y_Acc/1 -> WithoutRTK/9(GPS_Y_Acc), Multipath_detection/5(GPS_Y_Acc), RTK/12(GPS_Y_Acc)
  Unit Delay10/1 -> Multipath_detection/9(count_i)
  Multipath_detection/6(count_o) -> Unit Delay10/1

== system bus_roadtest_v3/RTI Data/RTI Data Store/RTI Data Store/RTI Data Store ==
  RTI Data Store : Subsystem  mask(RTI_DATA_STORE){}
      mask help:
      | RTI Data Store Block. This block is used by RTI to store internal model dependent data. Deleting this block will result in data loss.
      |
      | NEVER DELETE, COPY, OR MODIFY THIS BLOCK!
      mask Help:
      | RTI Data Store Block. This block is used by RTI to store internal model dependent data. Deleting this block will result in data loss.
      | 
      | NEVER DELETE, COPY, OR MODIFY THIS BLOCK!
      mask Display: text(0.5, 0.5, ' ', 'HorizontalAlignment', 'center');

== system bus_roadtest_v3/RTI Data/RTI Data Store/RTI Data Store/RTI Data Store/RTI Data Store ==

== matlab function bus_roadtest_v3/Target_planner/Boundingbox_trans ==
  data: OB_num output; V_boundingbox output; vehicle_state input
function [OB_num,V_boundingbox] = fcn(vehicle_state)

vehicle_x = vehicle_state(1);
vehicle_y = vehicle_state(2);
vehicle_heading = vehicle_state(3);

OB_num = 0;
V_boundingbox_vehicle = zeros(2,4);
V_boundingbox = V_boundingbox_vehicle;

for m = 1 : OB_num
    OBXY_m = V_boundingbox_vehicle(2*m-1:2*m,1:4);
    for i = 1 : 4
        V_boundingbox(2*m-1:2*m,i) = [cos(vehicle_heading),-sin(vehicle_heading);sin(vehicle_heading),cos(vehicle_heading)]*[OBXY_m(1,i);OBXY_m(2,i)]+[vehicle_x;vehicle_y];
    end
end

== matlab function bus_roadtest_v3/Positioning_module/ITRI_MM/UKF_Only/SLAM_UKF_MM_Check ==
  data: SLAM_op_dist input; SLAM_seg_LaneWidth input; MM_FaultFlag output; SLAM_seg_heading input; X_UKF_SLAM_heading input
function MM_FaultFlag = MMC(SLAM_op_dist,SLAM_seg_LaneWidth,SLAM_seg_heading,X_UKF_SLAM_heading)

MM_FaultFlag = 0;

if abs(SLAM_op_dist) > SLAM_seg_LaneWidth
    MM_FaultFlag = 1;
end
Heading_err = abs(SLAM_seg_heading - X_UKF_SLAM_heading);
if Heading_err > pi
    Heading_err = abs(2*pi - Heading_err);
end
if Heading_err > pi/4
    MM_FaultFlag = 1;
end

== matlab function bus_roadtest_v3/Data_RX/X-by-wire/Input_speed/Pulse_siganl_process ==
  data: update_flag output; duty input; freq_out output; freq input; duty_min input; duty_max input; freq_max input; rate_max input; Throttle_on input; freq_last input
function [update_flag,freq_out]  = fcn(duty,freq,duty_min,duty_max,freq_max,rate_max,Throttle_on,freq_last)

update_flag =1;

if(duty <= duty_min || duty >= duty_max) % duty ratio doesn't in the valid range
    update_flag = 0;
else
    if (freq > freq_max) || Throttle_on == 0 % freq exceed the max value
        update_flag = 0;
%     else
%         if (freq-freq_last > rate_max) % freq change rate exceed the max value
%             update_flag = 0;
%         end        
    end 
end

if (update_flag ==1)
    freq_out = freq;
else
    freq_out = freq_last;
end

== matlab function bus_roadtest_v3/Motion_controller/Longitudinal_control/Switching_module/Brake_Throttle_toggle ==
  data: B_toggle input; Brake_trig_CC output; T_toggle input; Last_status input; Static_flag input
function Brake_trig_CC = fcn(B_toggle,T_toggle,Last_status,Static_flag)
%#codegen
if Static_flag == 1
    Brake_trig_CC = ~Static_flag;
else
    if (B_toggle==0 && T_toggle ==0)
        Brake_trig_CC = Last_status;
    else
        Brake_trig_CC = B_toggle;
    end
end

== matlab function bus_roadtest_v3/Positioning_module/ITRI_MM/Check_New_SBG_and_x_y_coordination ==
  data: x output; y output; SBG_long input; SBG_lat input; SBG_alt input; SBG_Yaw input; REF_GPS_RFS input; z output; yaw_angle output
function [x,y,z,yaw_angle] = fcn(SBG_long,SBG_lat,SBG_alt,SBG_Yaw,REF_GPS_RFS)
%#codegen
[x,y,z] = dllh2denu(REF_GPS_RFS,[SBG_long,SBG_lat,SBG_alt]) ;
if 90-SBG_Yaw < 0
    yaw_angle = (90-SBG_Yaw+360)*pi/180;
else
    yaw_angle = (90-SBG_Yaw)*pi/180;
end
function [de,dn,du] =dllh2denu(llh0,llh)
%%% approximation version for GPS coordinate transformation from
%%% llh(longitude,latitude,altitude) to [de,dn,du]=(east,north,height) relatitive to a
%%% given reference point,llh0
% REF_GPS_RFS = [122.000000+20.0304416/60, 37.000000+54.8767679/60, 10.2266];  
% REF_GPS_RFS(1) = -REF_GPS_RFS(1); % Longitude: (-):West, (+):East

%%%%%constants
a = 6378137;
b = 6356752.3142;
e2 = 1 - (b/a)^2;
%%%%%% location of reference point in radians
phi = llh0(2)*pi/180;
lam = llh0(1)*pi/180;
h = llh0(3);
%%%%%%location of data points in radians
dphi = llh(:,2)*pi/180 - phi; % LATITUDE
dlam = llh(:,1)*pi/180 -lam;  % LONGITUDE
dh = llh(:,3)-h;  %altitude
%%%%%%% some useful definitions
tmp1 = sqrt(1-e2*sin(phi)^2);
% cl = cos(lam);
% sl = sin(lam);
cp = cos(phi);
sp = sin(phi);
%%%%%% Transformations
de = (a/tmp1+h)*cp*dlam- (a*(1-e2)/(tmp1^3)+h)*sp.*dphi.*dlam+cp.*dlam.*dh;
dn = (a*(1-e2)/tmp1^3+h)*dphi+1.5*cp*sp*a*e2*dphi.^2+sp^2.*dh.*dphi+0.5*sp*cp*(a/tmp1+h)*dlam.^2;
du = dh -0.5*(a-1.5*a*e2*cp^2+0.5*a*e2+h)*dphi.^2-0.5*cp^2*(a/tmp1-h)*dlam.^2;
%denu2 = [de,dn,du];
%%%%%%%%%%%%%%%%%%%%%%%%%%%

== matlab function bus_roadtest_v3/Motion_controller/Lateral_control/LKC_module/MATLAB Function ==
  data: current_cmd input; Cmd_rate input; final_cmd output; last_cmd input
function final_cmd = fcn(current_cmd,Cmd_rate,last_cmd)

if abs(current_cmd-last_cmd) < Cmd_rate
    final_cmd = current_cmd;
else
    final_cmd = sign(current_cmd-last_cmd) * Cmd_rate + last_cmd;
end

== matlab function bus_roadtest_v3/Positioning_module/ITRI_MM/UKF_Only/GNSS_Check/RTK ==
  data: GPS_update_True input; GNSS_FaultFlag_True input; GPS_X input; GPS_update output; GPS_Y input; GPS_Heading input; Road_Alt_GPS input; IMU_Sensor input; GPS_TYPE input; Last_GPS_Type_In input; X_UKF input; GPS_X_Acc input; GPS_Y_Acc input; Q_last_i input; R_last_i input; Last_GPS_In input; X_state output; GNSS_FaultFlag output; Q_last_o output; R_last_o output; Last_GPS_Out output; ResetP output; count_out output; count_in input; aaaaa output
function [GPS_update,X_state,GNSS_FaultFlag,Q_last_o,R_last_o,Last_GPS_Out,ResetP,count_out,aaaaa] = fcn(GPS_update_True,GNSS_FaultFlag_True,GPS_X,GPS_Y,GPS_Heading,Road_Alt_GPS,IMU_Sensor,GPS_TYPE,Last_GPS_Type_In,X_UKF,GPS_X_Acc,GPS_Y_Acc,Q_last_i,R_last_i,Last_GPS_In,count_in)

Last_X=Last_GPS_In(1);
Last_Y=Last_GPS_In(2);
Last_Heading = Last_GPS_In(3);
Sensor_Velocity = IMU_Sensor(1);
Sensor_Yawrate=IMU_Sensor(2);
Sensor_Grade=IMU_Sensor(3);

% if GPS_X==Last_X && GPS_Y==Last_Y || GPS_TYPE == 2
%     GPS_update = 0;
% else
%     GPS_update = 1;
% end
% if GPS_TYPE == 2
%     GPS_X_out = Last_X;
%     GPS_Y_out = Last_Y;
%     GPS_Heading_out = Last_Heading;
% else
%     GPS_X_out = GPS_X;
%     GPS_Y_out = GPS_Y;
%     GPS_Heading_out = GPS_Heading;    
% end  

ResetP = 0;
aaaaa = 0;

if GPS_update_True == 1
    count_out = 0;
else
    count_out = count_in;
end

dist_gpslastgps = sqrt((GPS_X-X_UKF(1))^2 + (GPS_Y-X_UKF(2))^2);
if dist_gpslastgps > 2
    GNSS_FaultFlag = 1;
else
    GNSS_FaultFlag = 0;
end
if GPS_X==Last_X && GPS_Y==Last_Y || GPS_TYPE == 2
    GPS_update = 0;
else
    if Sensor_Velocity >= 0.1 && dist_gpslastgps > 100
        GPS_update = 0;
    else
        GPS_update = 1;
    end
end

if GPS_X_Acc == 0
    GPS_X_Acc = 0.01;
end
if GPS_Y_Acc == 0
    GPS_Y_Acc = 0.01;
end

if abs(GPS_Heading - X_UKF(3)) > 5.5
    H_ACC = 100;
else
    H_ACC = 0.1;
end

if Sensor_Velocity >= 0.1
    if GPS_update == 0
        GPS_X_out = Last_X;
        GPS_Y_out = Last_Y;
        GPS_Heading_out = Last_Heading;
        Q = Q_last_i;
        R = R_last_i;
    else
        GPS_X_out = GPS_X;
        GPS_Y_out = GPS_Y;
        GPS_Heading_out = GPS_Heading;
        if GPS_TYPE == 7
            Q = diag([0.00025,0.00025,0.0000001,1,0.0001]);
            R = diag([GPS_X_Acc^2,GPS_Y_Acc^2,H_ACC,0.0001,0.0001]);
            if GPS_update_True == 1 && GNSS_FaultFlag_True == 1
                count_out = count_in + 1;
                if count_out == 1
%                     ResetP = 1;
                end
            end
        elseif GPS_TYPE == 6
            Q = diag([0.00025,0.00025,0.0000001,1,0.0001]);
            if GPS_X_Acc > 0.1 && GPS_Y_Acc > 0.1
                R = diag([GPS_X_Acc^2,GPS_Y_Acc^2,H_ACC,0.0001,0.0001]);
            else
                aaaaa = 1;
                if Last_GPS_Type_In == 6
                    R = R_last_i;
                else
                    R = diag([1,1,0.1,0.0001,0.0001]);
                end
            end
            if GPS_update_True == 1 && GNSS_FaultFlag_True == 1
                count_out = count_in + 1;
                if count_out == 1
%                     ResetP = 1;
                end
            end
        else
            Q = Q_last_i;
            R = R_last_i;
        end
    end
else
    if GPS_TYPE == 2
        GPS_X_out = Last_X;
        GPS_Y_out = Last_Y;
        GPS_Heading_out = Last_Heading;
    else
        GPS_X_out = GPS_X;
        GPS_Y_out = GPS_Y;
        GPS_Heading_out = GPS_Heading;
    end
    Q = diag([0.00025,0.00025,0.0000001,1,0.0001]);
    R = diag([GPS_X_Acc^2,GPS_Y_Acc^2,H_ACC,0.0001,0.0001]);
%     Q = diag([0.0001,0.0001,0.000001,1,0.0001,0.0001]);
%     R = diag([0.1,0.1,0.1,0.0005,0.0001,0.002]);
end

Q_last_o = Q;
R_last_o = R;

% if GPS_TYPE == 6 || GPS_TYPE == 7
%     if Last_GPS_Type_In == 2
%         ResetP = 1;
%     else
%         ResetP = 0;
%     end
% else
%     ResetP = 0;
% end

Last_GPS_Out = [GPS_X_out;GPS_Y_out;GPS_Heading_out];
X_state = [GPS_X_out,GPS_Y_out,GPS_Heading_out,Sensor_Yawrate,Sensor_Velocity]';

== matlab function bus_roadtest_v3/Flag_management/Fault detection/Fault detection(Control)/Brake fault detection/MATLAB Function1 ==
  settings: updateMethod=DISCRETE
  data: u input; y output
function y = my_average(u) %# codegen
persistent i buf bufSum;
if isempty(buf)
    buf = zeros(1,100); %averaging steps
    bufSum = 0;
    i = 1;
end
bufSum = bufSum - buf(i);
buf(i) = u;
bufSum = bufSum + u;
i = i + 1;
if i > numel(buf)
    i = 1;
end
y = bufSum / numel(buf);

== matlab function bus_roadtest_v3/Data_RX/SBG/MATLAB Function ==
  data: p_xy output; gps_long input; gps_lat input; REF_GPS_RFS input
function p_xy  = fcn(gps_long,gps_lat,REF_GPS_RFS)
%#codegen
[x,y,z] = dllh2denu(REF_GPS_RFS,[gps_long,gps_lat,29]) ;
p_xy=[x;y];



function [de,dn,du] =dllh2denu(llh0,llh)
%%% approximation version for GPS coordinate transformation from
%%% llh(longitude,latitude,altitude) to [de,dn,du]=(east,north,height) relatitive to a
%%% given reference point,llh0
% REF_GPS_RFS = [122.000000+20.0304416/60, 37.000000+54.8767679/60, 10.2266];  
% REF_GPS_RFS(1) = -REF_GPS_RFS(1); % Longitude: (-):West, (+):East

%%%%%constants
a = 6378137;
b = 6356752.3142;
e2 = 1 - (b/a)^2;
%%%%%% location of reference point in radians
phi = llh0(2)*pi/180;
lam = llh0(1)*pi/180;
h = llh0(3);
%%%%%%location of data points in radians
dphi = llh(:,2)*pi/180 - phi; % LATITUDE
dlam = llh(:,1)*pi/180 -lam;  % LONGITUDE
dh = llh(:,3)-h;  %altitude
%%%%%%% some useful definitions
tmp1 = sqrt(1-e2*sin(phi)^2);
% cl = cos(lam);
% sl = sin(lam);
cp = cos(phi);
sp = sin(phi);
%%%%%% Transformations
de = (a/tmp1+h)*cp*dlam- (a*(1-e2)/(tmp1^3)+h)*sp.*dphi.*dlam+cp.*dlam.*dh;
dn = (a*(1-e2)/tmp1^3+h)*dphi+1.5*cp*sp*a*e2*dphi.^2+sp^2.*dh.*dphi+0.5*sp*cp*(a/tmp1+h)*dlam.^2;
du = dh -0.5*(a-1.5*a*e2*cp^2+0.5*a*e2+h)*dphi.^2-0.5*cp^2*(a/tmp1-h)*dlam.^2;
%denu2 = [de,dn,du];
%%%%%%%%%%%%%%%%%%%%%%%%%%%

== matlab function bus_roadtest_v3/Data_TX/IPC/MATLAB Function ==
  data: Path_LV input; x1 output; y1 output; x2 output; y2 output; x3 output; y3 output; x4 output; y4 output; x5 output; y5 output; x6 output; y6 output
function [x1,y1,x2,y2,x3,y3,x4,y4,x5,y5,x6,y6] = fcn(Path_LV)

x1 = Path_LV(1,1);
y1 = Path_LV(2,1);
x2 = Path_LV(1,2);
y2 = Path_LV(2,2);
x3 = Path_LV(1,3);
y3 = Path_LV(2,3);
x4 = Path_LV(1,4);
y4 = Path_LV(2,4);
x5 = Path_LV(1,5);
y5 = Path_LV(2,5);
x6 = Path_LV(1,6);
y6 = Path_LV(2,6);

== matlab function bus_roadtest_v3/Positioning_module/ITRI_MM/Check_New_GPS_and_x_y_coordination ==
  data: x output; y output; gps_long input; gps_lat input; gps_alt input; yaw_rate input; Vt input; SBG_Course input; REF_GPS_RFS input; z output; yaw_rate1 output; yaw_angle output; u output
function [x,y,z,yaw_rate1,yaw_angle,u] = fcn(gps_long,gps_lat,gps_alt,yaw_rate,Vt,SBG_Course,REF_GPS_RFS)
%#codegen
[x,y,z] = dllh2denu(REF_GPS_RFS,[gps_long,gps_lat,gps_alt]) ;
yaw_rate1 = -yaw_rate;
if 90-SBG_Course < 0
    yaw_angle = (90-SBG_Course+360)*pi/180;
else
    yaw_angle = (90-SBG_Course)*pi/180;
end
u=[x;y;yaw_rate;Vt];
function [de,dn,du] =dllh2denu(llh0,llh)
%%% approximation version for GPS coordinate transformation from
%%% llh(longitude,latitude,altitude) to [de,dn,du]=(east,north,height) relatitive to a
%%% given reference point,llh0
% REF_GPS_RFS = [122.000000+20.0304416/60, 37.000000+54.8767679/60, 10.2266];  
% REF_GPS_RFS(1) = -REF_GPS_RFS(1); % Longitude: (-):West, (+):East

%%%%%constants
a = 6378137;
b = 6356752.3142;
e2 = 1 - (b/a)^2;
%%%%%% location of reference point in radians
phi = llh0(2)*pi/180;
lam = llh0(1)*pi/180;
h = llh0(3);
%%%%%%location of data points in radians
dphi = llh(:,2)*pi/180 - phi; % LATITUDE
dlam = llh(:,1)*pi/180 -lam;  % LONGITUDE
dh = llh(:,3)-h;  %altitude
%%%%%%% some useful definitions
tmp1 = sqrt(1-e2*sin(phi)^2);
% cl = cos(lam);
% sl = sin(lam);
cp = cos(phi);
sp = sin(phi);
%%%%%% Transformations
de = (a/tmp1+h)*cp*dlam- (a*(1-e2)/(tmp1^3)+h)*sp.*dphi.*dlam+cp.*dlam.*dh;
dn = (a*(1-e2)/tmp1^3+h)*dphi+1.5*cp*sp*a*e2*dphi.^2+sp^2.*dh.*dphi+0.5*sp*cp*(a/tmp1+h)*dlam.^2;
du = dh -0.5*(a-1.5*a*e2*cp^2+0.5*a*e2+h)*dphi.^2-0.5*cp^2*(a/tmp1-h)*dlam.^2;
%denu2 = [de,dn,du];
%%%%%%%%%%%%%%%%%%%%%%%%%%%

== matlab function bus_roadtest_v3/Speed_profile/High level controller/ACC/MATLAB Function1 ==
  data: cmd input; Ego_speed input; cmd_limited output
function cmd_limited = fcn(cmd, Ego_speed)
%#codegen
if cmd < (Ego_speed-5)
    cmd_limited = (Ego_speed-5);
else
    cmd_limited = cmd;
end

== matlab function bus_roadtest_v3/Data_RX/Xavier/MATLAB Function ==
  settings: updateMethod=DISCRETE
  data: PC input; PC_out output; RD input; PC_last input; count output
function [PC_out, count] = fcn(PC,RD,PC_last)
persistent counter
if isempty(counter)
    counter = 0;
end 
if abs(PC_last-PC)>5 
    if abs(RD-PC)<3 
        PC_out = PC;
        counter = 0;
    else
        PC_out = PC_last;
        counter = counter+1;
    end
else
    counter = 0;
    PC_out = PC;
end
count = counter;

== matlab function bus_roadtest_v3/Positioning_module/ITRI_MM/UKF_Only/Generate_sigma_pt_UKF ==
  data: IC_X input; X_AUG output; IC_P input; n input; gamma input
function X_AUG = fcn(IC_X,IC_P,n,gamma)
%#codegen
x0  = IC_X(:,1);
p0 = blkdiag(IC_P(:,1:5));
[p_sqrt,q]= chol(p0);
x_aug=zeros(5,11);

%% model 1
if q ~= 0; % p0 is not positive definite
%     disp('p0 is not positive definite');
    %Reset the covariance matrix by extracting the diagonal of original
    %covariance matrix p0 and check if any element is close to 0, which
    %can cause matrix singularity problem!
    temp_dia = abs(diag(p0));
    indcheck = find(temp_dia(:)<10^-10);
    if ~isempty(indcheck)
        temp_dia(indcheck) = 10^-10;
    end
    %p0 =diag(abs(diag(p0)));
    p0 = diag(temp_dia);
    
    %disp(p0);
    p_sqrt = chol(p0);
end

%%
p_sqrt = gamma.*(p_sqrt');

x_aug(:,1) = x0; %i = 0

for i = 1:n
    x_aug(:,i+1) = x0 + p_sqrt(:,i);
end

for i = 1:n
    x_aug(:,n+1+i) = x0 - p_sqrt(:,i);
end
X_AUG=[x_aug];
